simulink model "robotcontrol"  (R2022b)
settings: Solver=FixedStepAuto  StartTime=0.0  StopTime=10.0  RelTol=1e-3
libraries: vexarmcortexlib x14, vexcommonlib x2
settings Model: SimulationMode=external  ExtModeTrigDuration=25  Creator=robert  LastModifiedBy=robert
settings OptimizationCC: EnhancedBackFolding=on  PassReuseOutputArgsAs=Individual arguments  ZeroExternalMemoryAtStartup=off  ZeroInternalMemoryAtStartup=off  MaxStackSize=64  OptimizeBlockOrder=speed  DifferentSizesBufferReuse=on  OptimizationCustomize=off  EfficientTunableParamExpr=on
settings DebuggingCC: ParameterTunabilityLossMsg=error
settings HardwareCC: ProdBitPerPointer=32  ProdBitPerSizeT=32  ProdBitPerPtrDiffT=32  ProdLargestAtomicInteger=Long  ProdLargestAtomicFloat=Double  ProdWordSize=32  ProdHWDeviceType=ARM Compatible->ARM Cortex  UseEmbeddedCoderFeatures=off
settings SFSimCC: MATLABDynamicMemAlloc=off
settings RTWCC: Description=Embedded Coder  SystemTargetFile=ert.tlc  HardwareBoard=ARM Cortex-based VEX Microcontroller  TLCOptions="-aInlineSetEventsForThisBaseRateFcn=TLC_FALSE -aSuppressMultiTaskScheduler=TLC_FALSE  -aRateBasedStepFcn=0"  TemplateMakefile=ert_default_tmf  Toolchain=GNU Tools for VEX ARM Cortex
settings CodeAppCC: ForceParamTrailComments=on  IgnoreCustomStorageClasses=off  OperatorAnnotations=on  SimulinkDataObjDesc=on  SFDataObjDesc=on  InsertBlockDesc=on
settings ERTTargetCC: SupportNonInlinedSFcns=on  ExtModeTransport=1  ExtModeMexFile=ext_serial_win32_comm

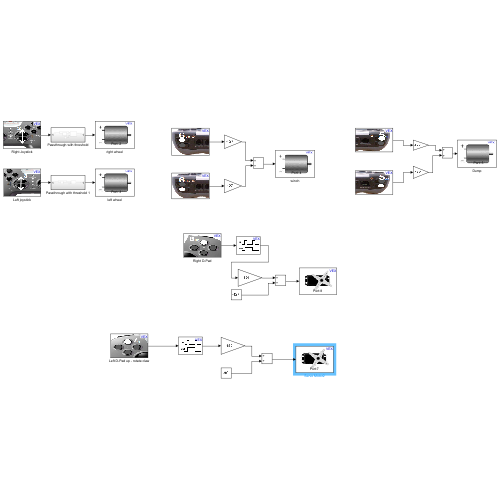
[thumbnail: Simulink's stored preview of the top-level diagram]
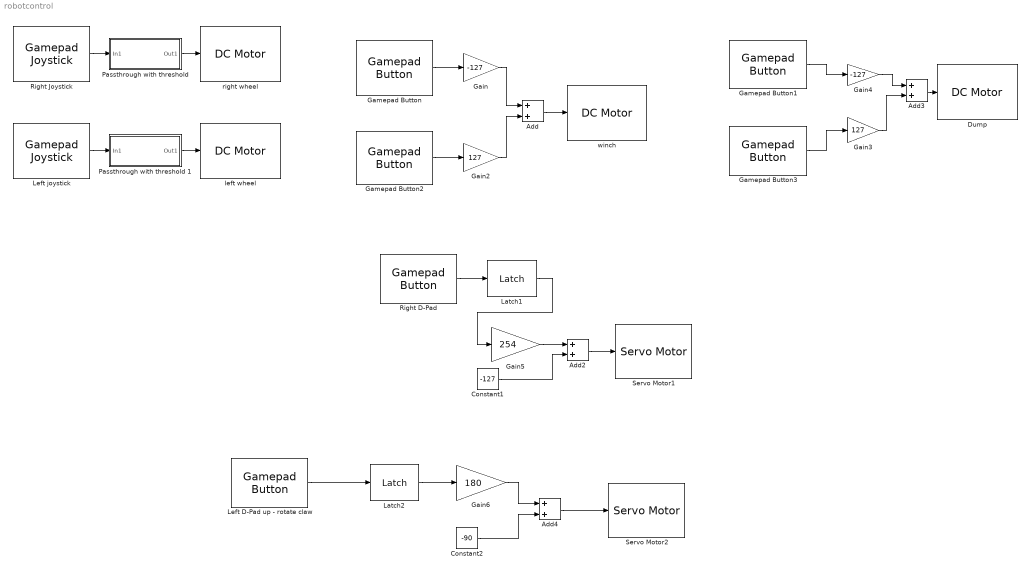
== system robotcontrol ==
  Add{,2..4} (4 alike) : Sum
  Constant1 : Constant  Value=-127
  Constant2 : Constant  Value=-90
  Dump : vexarmcortexlib/Actuators/DC Motor  motor=5  scaleFactor=1/13.5  SimulationOut=off
  Gain : Gain  Gain=-127
  Gain2 : Gain  Gain=127
  Gain3 : Gain  Gain=127
  Gain4 : Gain  Gain=-127
  Gain5 : Gain  Gain=254
  Gain6 : Gain  Gain=180
  Gamepad Button : vexarmcortexlib/Gamepad/Gamepad Button  joystick=1  chan=6  button56=Up  button78=Down  SimulationIn=off  SampleTime=0.02
  Gamepad Button1 : vexarmcortexlib/Gamepad/Gamepad Button  joystick=1  chan=5  button56=Up  button78=Down  SimulationIn=off  SampleTime=0.02
  Gamepad Button2 : vexarmcortexlib/Gamepad/Gamepad Button  joystick=1  chan=6  button56=Down  button78=Down  SimulationIn=off  SampleTime=0.02
  Gamepad Button3 : vexarmcortexlib/Gamepad/Gamepad Button  joystick=1  chan=5  button56=Down  button78=Down  SimulationIn=off  SampleTime=0.02
  Latch1 : vexcommonlib/Latch  output0=off  BlockPlatform=vexarmcortex
      settings: LibrarySourceBlock=vexarmcortexlib/Utilities/Latch
  Latch2 : vexcommonlib/Latch  output0=off  BlockPlatform=vexarmcortex
      settings: LibrarySourceBlock=vexarmcortexlib/Utilities/Latch
  Left D-Pad up - rotate claw : vexarmcortexlib/Gamepad/Gamepad Button  joystick=1  chan=7  button56=Up  button78=Up  SimulationIn=off  SampleTime=0.02
  Left joystick : vexarmcortexlib/Gamepad/Gamepad Joystick  joystick=1  chan=3  SimulationIn=off  SampleTime=0.02
  Passthrough with threshold : Subsystem
  Passthrough with threshold 1 : Subsystem
  Right D-Pad : vexarmcortexlib/Gamepad/Gamepad Button  joystick=1  chan=8  button56=Up  button78=Up  SimulationIn=off  SampleTime=0.02
  Right Joystick : vexarmcortexlib/Gamepad/Gamepad Joystick  joystick=1  chan=2  SimulationIn=off  SampleTime=0.02
  Servo Motor1 : vexarmcortexlib/Actuators/Servo Motor  motor=8  scaleFactor=60/127  SimulationOut=off
  Servo Motor2 : vexarmcortexlib/Actuators/Servo Motor  motor=7  scaleFactor=60/127  SimulationOut=off
  left wheel : vexarmcortexlib/Actuators/DC Motor  motor=3  scaleFactor=1/13.5  SimulationOut=off
  right wheel : vexarmcortexlib/Actuators/DC Motor  motor=2  scaleFactor=1/13.5  SimulationOut=off
  winch : vexarmcortexlib/Actuators/DC Motor  motor=4  scaleFactor=1/13.5  SimulationOut=off
  wires:
  Gamepad Button/1 -> Gain/1
  Gamepad Button2/1 -> Gain2/1
  Gain/1 -> Add/1
  Gain2/1 -> Add/2
  Add/1 -> winch/1
  Left joystick/1 -> Passthrough with threshold 1/1(In1)
  Right Joystick/1 -> Passthrough with threshold/1(In1)
  Passthrough with threshold 1/1(Out1) -> left wheel/1
  Passthrough with threshold/1(Out1) -> right wheel/1
  Gamepad Button3/1 -> Gain3/1
  Gamepad Button1/1 -> Gain4/1
  Add3/1 -> Dump/1
  Gain4/1 -> Add3/1
  Gain3/1 -> Add3/2
  Gain5/1 -> Add2/1
  Right D-Pad/1 -> Latch1/1
  Latch1/1 -> Gain5/1
  Add2/1 -> Servo Motor1/1
  Constant1/1 -> Add2/2
  Constant2/1 -> Add4/2
  Latch2/1 -> Gain6/1
  Left D-Pad up - rotate claw/1 -> Latch2/1
  Add4/1 -> Servo Motor2/1
  Gain6/1 -> Add4/1

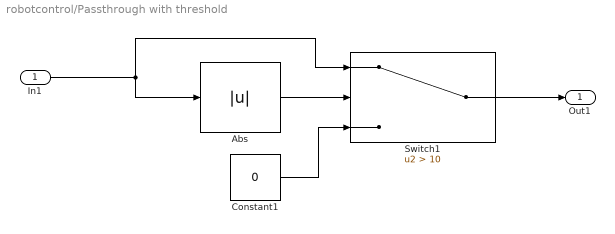
== system robotcontrol/Passthrough with threshold ==
  In1 : Inport
  Abs : Abs  SaturateOnIntegerOverflow=off
  Constant1 : Constant  Value=0
  Switch1 : Switch  Criteria=u2 > Threshold  Threshold=10  SaturateOnIntegerOverflow=off  InputSameDT=off
  Out1 : Outport
  wires:
  Constant1/1 -> Switch1/3
  Abs/1 -> Switch1/2
  Switch1/1 -> Out1/1
  In1/1 -> Abs/1, Switch1/1

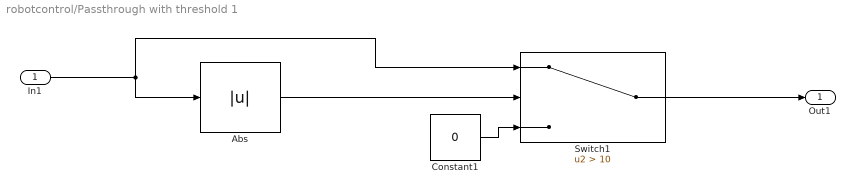
== system robotcontrol/Passthrough with threshold 1 ==
  In1 : Inport
  Abs : Abs  SaturateOnIntegerOverflow=off
  Constant1 : Constant  Value=0
  Switch1 : Switch  Criteria=u2 > Threshold  Threshold=10  SaturateOnIntegerOverflow=off  InputSameDT=off
  Out1 : Outport
  wires:
  Constant1/1 -> Switch1/3
  Abs/1 -> Switch1/2
  Switch1/1 -> Out1/1
  In1/1 -> Abs/1, Switch1/1
